simulink model "iC_1ph_MR2_0829"  (Simulink 7.5)
settings: Solver=ode14x  StartTime=0.0  StopTime=30/60  FixedStep=Ts1  RelTol=1e-3
PostLoadFcn:
  | , if any(exist('dsrtsu_mdlpostloadfcn', 'file') == [2, 3, 6]), try dsrtsu_mdlpostloadfcn('Execute', bdroot); catch fprintf('Error in PostLoadFcn (dsrtsu_mdlpostloadfcn) for model "%s":\n %s\n', bdroot, lasterr); end, end,
InitFcn:
  | iC_ini
values from neighbouring files (symbols this model uses):
  C = Cideal+deltaC    (= 4e-05)    [IMC_calculo_limites_thetas.m]    (also in IMC_ini.m; JORGE_controlador_LCL_malha_interna.m; LCL_PAPM.m; R_in_LCL.m)
  excitacao_persistente = 0    [iC_ini.m]    (also in vC_ini.m)
  flag_time = 60/60    (= 1)    [iC_ini.m]    (also in vC_ini.m)
  init_time = 60/60    (= 1)    [iC_ini.m]
  L1 = L1ideal+deltaL1    (= 0.002)    [IMC_calculo_limites_thetas.m]    (also in IMC_ini.m; LCL_PAPM.m; R_in_LCL.m; calculo_FTs.m)
  L2 = L2ideal+deltaL2+Lgideal+deltaLg    (= 0.002)    [IMC_calculo_limites_thetas.m]    (also in IMC_ini.m; LCL_PAPM.m; R_in_LCL.m; calculo_FTs.m)
  param_change_time = 60/60    (= 1)    [iC_ini.m]    (also in vC_ini.m = 10)
  R1 = R1ideal+deltaR1    (= 1)    [IMC_calculo_limites_thetas.m]    (also in IMC_ini.m; R_in_LCL.m = 0; gera_resultados.m = 0; iC_ini.m = 0)
  R2 = R2ideal+deltaR2+Rgideal+deltaRg    (= 1)    [IMC_calculo_limites_thetas.m]    (also in IMC_ini.m; R_in_LCL.m = 0; gera_resultados.m = 0; iC_ini.m = 0)
  R_init = 10    [iC_ini.m]
  ref_phaseInv_time = 60/60    (= 1)    [iC_ini.m]    (also in vC_ini.m = 3.33333333333)
  ref_step_time = 60/60    (= 1)    [iC_ini.m]    (also in vC_ini.m = 6.66666666667)
  Ts = 1/12000    (= 8.33333333333e-05)    [IMC_calculo_limites_thetas.m]    (also in IMC_datta_ini.m = 0.5; IMC_ini.m; JORGE_controlador_LCL_malha_interna.m; LCL_PAPM.m)
  Ts1 = Ts/10    (= 8.33333333333e-06)    [iC_ini.m]    (also in vC_ini.m = 8.33333333333e-08)
  VCC = 1700    [iC_ini.m]    (also in vC_ini.m = 1200)
libraries: powerlib x14, powerlib_extras x1
settings Model: DSRTSU_INTERNAL_RTI_VER=390  DSRTSU_INTERNAL_RTI_TYPE=rti1103  Creator=dpbernardon  LastModifiedBy=dpbernardon  BufferReuse=off
settings SolverCC: AutoInsertRateTranBlk=on
settings OptimizationCC: BlockReduction=off  OptimizeBlockIOStorage=off  BufferReuse=off  ExpressionFolding=off  LocalBlockOutputs=off
settings HardwareCC: ProdIntDivRoundTo=Zero  ProdEndianess=BigEndian  ProdHWDeviceType=Generic->Custom  TargetIntDivRoundTo=Zero  TargetEndianess=BigEndian  TargetHWDeviceType=Generic->Custom
settings RTWCC: SystemTargetFile=rti1103.tlc  MakeCommand=make_rti  TemplateMakefile=rti1103.tmf  Description=dSPACE DS1103 Hardware Platform  ProcessScript=rti1103_make_rtw_hook
settings STFCustomTargetCC: ParMdlRefBuildCompliant=on  GeneratePreprocessorConditionals=Disable all  MatFileLogging=on  SystemTargetFile=rti1103.tlc
settings GRTTargetCC: CompOptLevelCompliant=off  ExtModeMexFile=noextcomm
settings CustomProperty: DataType=RTWOptions_EnumType_C__dSPACE RCPHIL 72_matlab_rti1103_tlc_rti1103_1InitialSimState  Value=RUN
settings EnumStrPairs: String=RUN

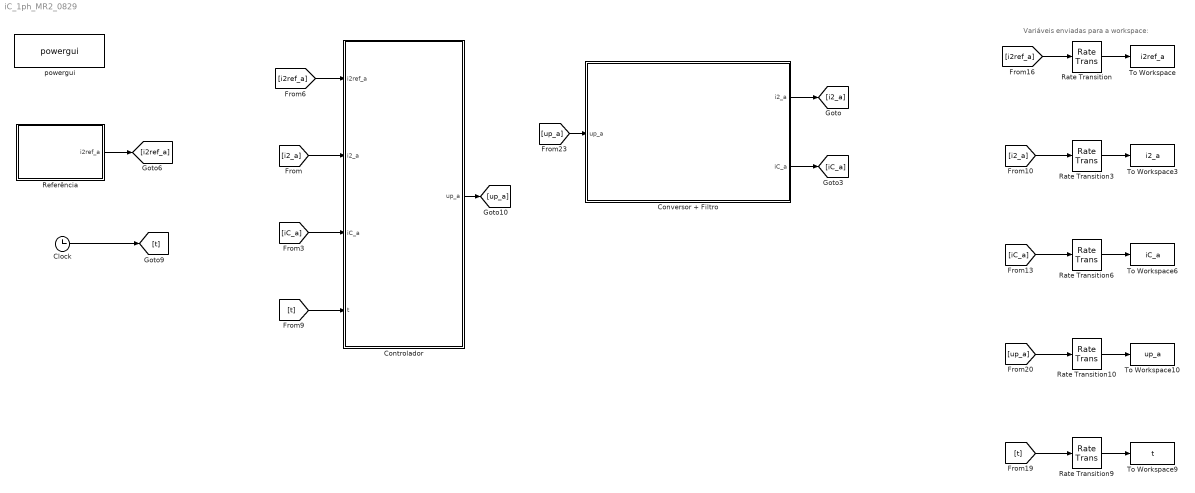
== system iC_1ph_MR2_0829 ==
  note: Variáveis enviadas para a workspace:
  Clock : Clock
      settings: Decimation=10
  Controlador : Subsystem
  Conversor + Filtro : Subsystem
  Rate Transition{,3,6,9..10} (5 alike) : RateTransition  OutPortSampleTime=Ts1
  Referência : Subsystem
  To Workspace : ToWorkspace  VariableName=i2ref_a  SampleTime=Ts1  SaveFormat=Array
  To Workspace10 : ToWorkspace  VariableName=up_a  SampleTime=Ts1  SaveFormat=Array
  To Workspace3 : ToWorkspace  VariableName=i2_a  SampleTime=Ts1  SaveFormat=Array
  To Workspace6 : ToWorkspace  VariableName=iC_a  SampleTime=Ts1  SaveFormat=Array
  To Workspace9 : ToWorkspace  VariableName=t  SampleTime=Ts1  SaveFormat=Array
  powergui : powerlib/powergui  Priority=1  SystemSampleTime=-1  SimulationMode=Discrete  SampleTime=Ts1  frequency=60  SPID=off  DisableSnubberDevices=off  DisableRonSwitches=off  DisableVfSwitches=off  SwTol=0  Interpol=off  frequencyindice=0  echomessages=off  HookPort=off  DisplayEquations=off  FunctionMessages=off  EnableUseOfTLC=off  x0status=blocks  RestoreLinks=warning  ResistiveCurrentMeasurement=off  Frange=[0:2:500]  Ylog=off  Xlog=on  ShowGrid=off  save=off  variable=ZData  ZoomFFT=off  StartTime=0.0  cycles=1  DisplayStyle=1  fundamental=60  FreqAxis=off  MaxFrequency=1000  frequencyindicesteady=1  RmsSteady=1  display=off  Ts=0  methode=off
  wires:
  Conversor + Filtro/1(i2_a) -> [i2_a]
  Conversor + Filtro/2(iC_a) -> [iC_a]
  [i2_a] -> Controlador/2(i2_a)
  [iC_a] -> Controlador/3(iC_a)
  Referência/1(i2ref_a) -> [i2ref_a]
  [i2ref_a] -> Controlador/1(i2ref_a)
  Clock/1 -> [t]
  [t] -> Controlador/4(t)
  [i2ref_a] -> Rate Transition/1
  [i2_a] -> Rate Transition3/1
  [iC_a] -> Rate Transition6/1
  [t] -> Rate Transition9/1
  Rate Transition/1 -> To Workspace/1
  Rate Transition3/1 -> To Workspace3/1
  Rate Transition6/1 -> To Workspace6/1
  Rate Transition9/1 -> To Workspace9/1
  [up_a] -> Rate Transition10/1
  Rate Transition10/1 -> To Workspace10/1
  Controlador/1(up_a) -> [up_a]
  [up_a] -> Conversor + Filtro/1(up_a)

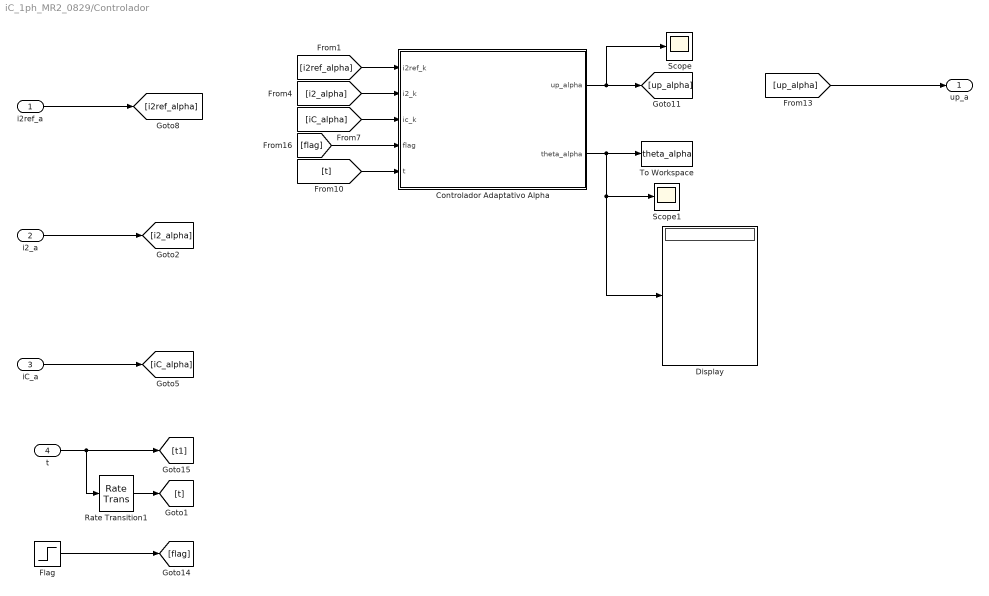
== system iC_1ph_MR2_0829/Controlador ==
  i2ref_a : Inport
  i2_a : Inport  Port=2
  iC_a : Inport  Port=3
  t : Inport  Port=4
  Controlador Adaptativo Alpha : Stateflow chart  TreatAsAtomicUnit=on  SystemSampleTime=Ts
      settings: MinAlgLoopOccurrences=on  RTWSystemCode=Function
  Display : Display
  Flag : Step  Time=flag_time  Before=1  After=0  SampleTime=Ts
  Rate Transition1 : RateTransition  OutPortSampleTime=Ts
  Scope : Scope
      settings: YMin=-5500  YMax=5000  SaveName=ScopeData4
  Scope1 : Scope
      settings: YMin=-5500  YMax=5000
  To Workspace : ToWorkspace  VariableName=theta_alpha  SampleTime=Ts1  SaveFormat=Array
  up_a : Outport
  wires:
  t/1 -> Rate Transition1/1, [t1]
  Rate Transition1/1 -> [t]
  i2_a/1 -> [i2_alpha]
  iC_a/1 -> [iC_alpha]
  [i2ref_alpha] -> Controlador Adaptativo Alpha/1(i2ref_k)
  [i2_alpha] -> Controlador Adaptativo Alpha/2(i2_k)
  [iC_alpha] -> Controlador Adaptativo Alpha/3(ic_k)
  [t] -> Controlador Adaptativo Alpha/5(t)
  Controlador Adaptativo Alpha/1(up_alpha) -> [up_alpha], Scope/1
  [up_alpha] -> up_a/1
  Flag/1 -> [flag]
  [flag] -> Controlador Adaptativo Alpha/4(flag)
  Controlador Adaptativo Alpha/2(theta_alpha) -> To Workspace/1, Scope1/1, Display/1
  i2ref_a/1 -> [i2ref_alpha]

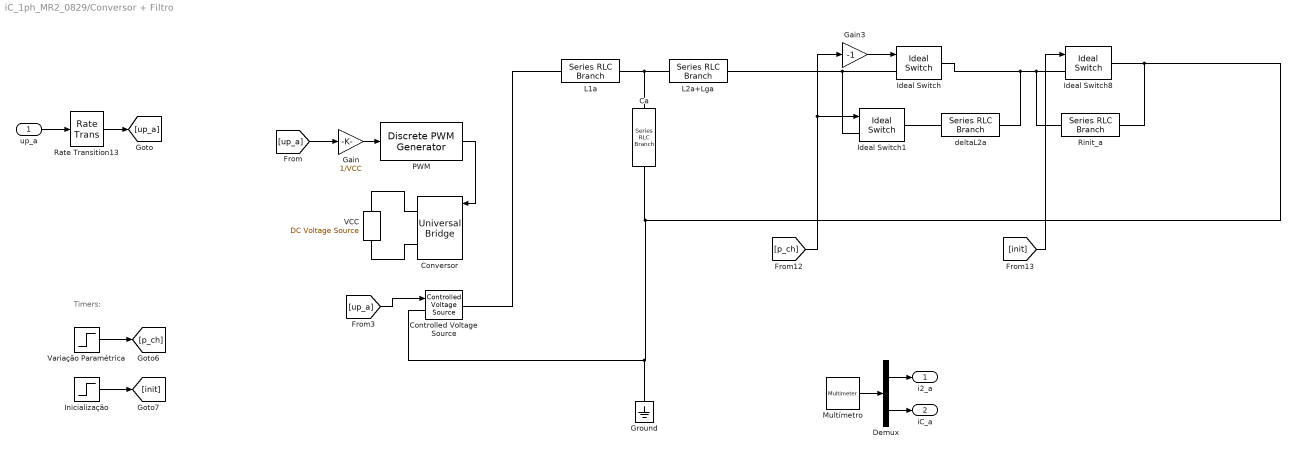
== system iC_1ph_MR2_0829/Conversor + Filtro ==
  note: Timers:
  up_a : Inport
  Ca : powerlib/Elements/Series RLC Branch  DialogController=POWERSYS.PowerSysDialog  PhysicalDomain=powersysdomain  SubClassName=unknown  LeftPortType=p1  RightPortType=p1  LConnTagsString=__new0  RConnTagsString=__new0  BranchType=C  Resistance=1  Inductance=1e-3  SetiL0=off  InitialCurrent=0  Capacitance=C  Setx0=off  InitialVoltage=0  Measurements=Branch current
  Controlled Voltage Source : powerlib/Electrical Sources/Controlled Voltage Source  DialogController=POWERSYS.PowerSysDialog  SystemSampleTime=-1  Initialize=on  Source_Type=AC  Amplitude=0  Phase=0  Frequency=0  Measurements=None
  Conversor : powerlib/Power Electronics/Universal Bridge  DialogController=POWERSYS.PowerSysDialog  SystemSampleTime=-1  Arms=3  SnubberResistance=1e5  SnubberCapacitance=inf  Device=IGBT / Diodes  Ron=1e-3  Lon=0  ForwardVoltages="[  0  0  ]"  ForwardVoltage=0  GTOparameters=[ 10e-6 , 20e-6 ]  IGBTparameters=[ 1e-6 , 2e-6 ]  Measurements=UAB UBC UCA UDC voltages  Measurements_2=None  converterType=Rectifier
  Demux : Demux  Outputs=2
  Gain : Gain  Gain=1/VCC  SampleTime=Ts1
  Gain3 : Gain  Gain=-1  SampleTime=Ts1
  Ground : powerlib/Elements/Ground  DialogController=POWERSYS.PowerSysDialog  PhysicalDomain=powersysdomain  SubClassName=unknown  LeftPortType=p1  RightPortType=p1  LConnTagsString=a
  Ideal Switch : powerlib/Power Electronics/Ideal Switch  DialogController=POWERSYS.PowerSysDialog  SystemSampleTime=-1  Ron=0.001  Lon=0  IC=1  Rs=1e5  Cs=inf  Measurements=off
  Ideal Switch1 : powerlib/Power Electronics/Ideal Switch  DialogController=POWERSYS.PowerSysDialog  SystemSampleTime=-1  Ron=0.001  Lon=0  IC=0  Rs=1e5  Cs=inf  Measurements=off
  Ideal Switch8 : powerlib/Power Electronics/Ideal Switch  DialogController=POWERSYS.PowerSysDialog  SystemSampleTime=-1  Ron=0.001  Lon=0  IC=1  Rs=1e5  Cs=inf  Measurements=off
  Inicialização : Step  Time=init_time  Before=1  After=0  SampleTime=Ts1
  L1a : powerlib/Elements/Series RLC Branch  DialogController=POWERSYS.PowerSysDialog  PhysicalDomain=powersysdomain  SubClassName=unknown  LeftPortType=p1  RightPortType=p1  LConnTagsString=__new0  RConnTagsString=__new0  BranchType=RL  Resistance=R1  Inductance=L1  SetiL0=off  InitialCurrent=0  Capacitance=1e-6  Setx0=off  InitialVoltage=0  Measurements=Branch current
  L2a+Lga : powerlib/Elements/Series RLC Branch  DialogController=POWERSYS.PowerSysDialog  PhysicalDomain=powersysdomain  SubClassName=unknown  LeftPortType=p1  RightPortType=p1  LConnTagsString=__new0  RConnTagsString=__new0  BranchType=RL  Resistance=R2  Inductance=L2  SetiL0=off  InitialCurrent=0  Capacitance=1e-6  Setx0=off  InitialVoltage=0  Measurements=Branch current
  Multímetro : powerlib/Measurements/Multimeter  SystemSampleTime=-1  PhasorSimulation=off  OutputType=Complex  sel=[7 5]  L=7  Gain=[1 1]  yselected={'Ib: Conversor + Filtro/L2a+Lga','Ib: Conversor + Filtro/Ca'};  PSBOutputType=1  PSBequivalent=0  AxesSetting=[0,0.1,-100,100]  Display=0  SavedBlockNames=-11
  PWM : powerlib_extras/Discrete  Control Blocks/Discrete PWM Generator  DialogController=POWERSYS.PowerSysDialog  SystemSampleTime=-1  GeneratorMode="3-arm  bridge (6 pulses)"  Fc=12000  Ts=Ts1  Internal=off  mIndex=0.4  Freq=60  Phase=0
  Rate Transition13 : RateTransition  OutPortSampleTime=Ts1
  Rinit_a : powerlib/Elements/Series RLC Branch  DialogController=POWERSYS.PowerSysDialog  PhysicalDomain=powersysdomain  SubClassName=unknown  LeftPortType=p1  RightPortType=p1  LConnTagsString=__new0  RConnTagsString=__new0  BranchType=RL  Resistance=R_init  Inductance=5*L2  SetiL0=off  InitialCurrent=0  Capacitance=1e-6  Setx0=off  InitialVoltage=0  Measurements=None
  VCC : powerlib/Electrical Sources/DC Voltage Source  DialogController=POWERSYS.PowerSysDialog  SystemSampleTime=-1  Amplitude=VCC  Measurements=None
  Variação Paramétrica : Step  Time=param_change_time  Before=-1  SampleTime=Ts1
  deltaL2a : powerlib/Elements/Series RLC Branch  DialogController=POWERSYS.PowerSysDialog  PhysicalDomain=powersysdomain  SubClassName=unknown  LeftPortType=p1  RightPortType=p1  LConnTagsString=__new0  RConnTagsString=__new0  BranchType=RL  Resistance=0  Inductance=5*L2  SetiL0=off  InitialCurrent=0  Capacitance=1e-6  Setx0=off  InitialVoltage=0  Measurements=None
  i2_a : Outport
  iC_a : Outport  Port=2
  wires:
  Gain/1 -> PWM/1
  up_a/1 -> Rate Transition13/1
  Rate Transition13/1 -> [up_a]
  PWM/1 -> Conversor/1
  [up_a] -> Gain/1
  [up_a] -> Controlled Voltage Source/1
  Multímetro/1 -> Demux/1
  Demux/1 -> i2_a/1
  Variação Paramétrica/1 -> [p_ch]
  Gain3/1 -> Ideal Switch/1
  [init] -> Ideal Switch8/1
  Inicialização/1 -> [init]
  [p_ch] -> Gain3/1, Ideal Switch1/1
  Demux/2 -> iC_a/1
  connections:
  Ideal Switch/RConn1 -- deltaL2a/RConn1 -- Ideal Switch8/LConn1 -- Rinit_a/LConn1
  Ca/LConn1 -- L2a+Lga/LConn1 -- L1a/RConn1
  Conversor/RConn1 -- VCC/RConn1
  VCC/LConn1 -- Conversor/RConn2
  L2a+Lga/RConn1 -- Ideal Switch/LConn1 -- Ideal Switch1/LConn1
  deltaL2a/LConn1 -- Ideal Switch1/RConn1
  Rinit_a/RConn1 -- Ideal Switch8/RConn1 -- Ground/LConn1 -- Controlled Voltage Source/LConn1 -- Ca/RConn1
  Controlled Voltage Source/RConn1 -- L1a/LConn1

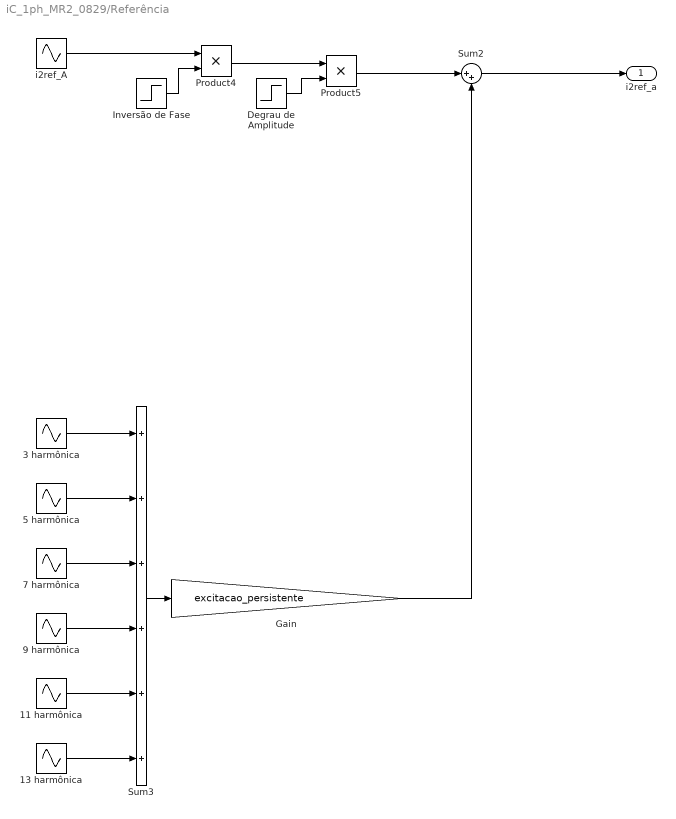
== system iC_1ph_MR2_0829/Referência ==
  11 harmônica : Sin  Amplitude=1.2  Bias=0  Frequency=2*pi*60*11  Phase=0  Samples=10  SampleTime=Ts  Offset=0
  13 harmônica : Sin  Amplitude=1.2  Bias=0  Frequency=2*pi*60*13  Phase=0  Samples=10  SampleTime=Ts  Offset=0
  3 harmônica : Sin  Amplitude=1.2  Bias=0  Frequency=2*pi*60*3  Phase=0  Samples=10  SampleTime=Ts  Offset=0
  5 harmônica : Sin  Amplitude=1.2  Bias=0  Frequency=2*pi*60*5  Phase=0  Samples=10  SampleTime=Ts  Offset=0
  7 harmônica : Sin  Amplitude=1.2  Bias=0  Frequency=2*pi*60*7  Phase=0  Samples=10  SampleTime=Ts  Offset=0
  9 harmônica : Sin  Amplitude=1.2  Bias=0  Frequency=2*pi*60*9  Phase=0  Samples=10  SampleTime=Ts  Offset=0
  Degrau de Amplitude : Step  Time=ref_step_time  Before=1  After=2  SampleTime=Ts
  Gain : Gain  Gain=excitacao_persistente  SampleTime=Ts
  Inversão de Fase : Step  Time=ref_phaseInv_time  Before=1  After=-1  SampleTime=Ts
  Product4 : Product  SampleTime=Ts  RndMeth=Zero
  Product5 : Product  SampleTime=Ts  RndMeth=Zero
  Sum2 : Sum  Inputs=|++
  Sum3 : Sum  Inputs=++++++
  i2ref_A : Sin  Amplitude=2  Bias=0  Frequency=2*pi*60  Phase=0  Samples=10  SampleTime=Ts  Offset=0
  i2ref_a : Outport
  wires:
  Product4/1 -> Product5/1
  Inversão de Fase/1 -> Product4/2
  Degrau de Amplitude/1 -> Product5/2
  i2ref_A/1 -> Product4/1
  Product5/1 -> Sum2/1
  Gain/1 -> Sum2/2
  Sum2/1 -> i2ref_a/1
  3 harmônica/1 -> Sum3/1
  5 harmônica/1 -> Sum3/2
  7 harmônica/1 -> Sum3/3
  9 harmônica/1 -> Sum3/4
  11 harmônica/1 -> Sum3/5
  13 harmônica/1 -> Sum3/6
  Sum3/1 -> Gain/1

== matlab function Controlador/Controlador Adaptativo Alpha ==
  data: i2ref_k input double; up_alpha output double; i2_k input double; ic_k input double; flag input double; t input double; theta_alpha output double
function [up_alpha,theta_alpha] = adaptativo( i2ref_k, i2_k, ic_k, flag, t )

%#CODEGEN
    
%Definição dos valores projetados dos elementos do filtro
L1ideal=2e-3;
L2ideal=2e-3;
Lgideal=0;
Cideal=40e-6;
R1ideal=0;
R2ideal=0;
Rgideal=0;

%Definição de erros percentuais para simular variação paramétrica
errL1=0;
errL2=0;
errLg=0;
errC=0;
errR1=0;
errR2=0;
errRg=0;
deltaL1=errL1*L1ideal;
deltaL2=errL2*L2ideal;
deltaLg=errLg*Lgideal;
deltaC=errC*Cideal;
deltaR1=errR1*R1ideal;
deltaR2=errR2*R2ideal;
deltaRg=errRg*Rgideal;

%Definição do valor real medido, incluindo a variação paramétrica
%percentual
L1=L1ideal+deltaL1;
L2=L2ideal+deltaL2+Lgideal+deltaLg;
C=Cideal+deltaC;
R1=R1ideal+deltaR1;
R2=R2ideal+deltaR2+Rgideal+deltaRg;

%Demais elementos
Ts=1/12000;
w=sqrt((L1+L2)/(L1*L2*C));

%Kp é a multiplicação do ganho do controlador da malha interna(kp), do
%ganho da planta(ki) e do ganho da malha externa(kod)
kp=8;
%Kp=0.156891976007044;
Kp=0.004780841242217;

%polos do modelo de referência:
p1=0.2;
p2=0.2;

km=(1-p1)*(1-p2);

%constantes -> gamaD < (1-gama)*km/kp
gamaD=0.0098;
gama=0.99;

delta0=0.8;

%adapt_time=2/60;
%vg_switch_time=4/60;

%if t>=19/60
%    stop=1;
%end

%% Variáveis Persistentes e Inicializações

persistent theta_k;
if isempty(theta_k)
    %COM compensação para vg
    %theta_k=[-0.3106; -0.2728; 0.0368; -0.2369; -0.422; -0.2775; -0.7979; 1.786; -0.0008; 0.0003];
    %theta_k=[-0.3106; -0.2728; 0.0368; -0.2369; -0.422; -0.2775; -0.7979; 1.786; 1; 0];
    %theta_k=[-0.40085038; -0.36853743; -0.064251891; -0.4277604154; -0.61214672; -0.46675405; -0.98929343; 1.76426551; 0.17164080; 0.11598547];
    %theta_k=[0;0;0;0;0;0; -0.98929343; 1.76426551; 0.17164080; 0.11598547];
    %theta_k=[-0.071151848470510; -0.470549298500393; -0.993323557655345; 1.762541193804541; 0.118014567931226; 0.108368323169129];
    %theta_k=[-0.46; -0.58; -1.74; 1.73; 0.2; 0.03];
    %theta_k=[-0.03; -0.36; -0.57; -0.01; 0.16; 0.02];
    theta_k=[0.34; -0.36; -0.51; 0.86; 0; 0];
end

persistent omega_k;
if isempty(omega_k)
    %COM vg
    omega_k=[0; 0; 0; 0; 0; 0];
end

persistent omega_k_1;
if isempty(omega_k_1)
    %COM vg
    omega_k_1=[0; 0; 0; 0; 0; 0];
end

persistent omega_k_2;
if isempty(omega_k_2)
    %COM vg
    omega_k_2=[0; 0; 0; 0; 0; 0];
end

%persistent omega_k_3;
%if isempty(omega_k_3)
%    %COM vg
%    omega_k_3=[0; 0; 0; 0; 0; 0];
%end

persistent eta_k_1;
if isempty(eta_k_1)
    %COM vg
    eta_k_1=[0; 0; 0; 0; 0; 0];
end

persistent eta_k_2;
if isempty(eta_k_2)
    %COM vg
    eta_k_2=[0; 0; 0; 0; 0; 0];
end

%persistent eta_k_3;
%if isempty(eta_k_3)
%    %COM vg
%    eta_k_3=[0; 0; 0; 0; 0; 0];
%end

persistent i2m_k_1;
if isempty(i2m_k_1)
    i2m_k_1=0;
end

persistent i2m_k_2;
if isempty(i2m_k_2)
    i2m_k_2=0;
end

%persistent i2m_k_3;
%if isempty(i2m_k_3)
%    i2m_k_3=0;
%end

persistent i2ref_k_1;
if isempty(i2ref_k_1)
    i2ref_k_1=0;
end

persistent i2ref_k_2;
if isempty(i2ref_k_2)
    i2ref_k_2=0;
end

%persistent i2ref_k_3;
%if isempty(i2ref_k_3)
%    i2ref_k_3=0;
%end

persistent v_k_1;
if isempty(v_k_1)
    v_k_1=0;
end

persistent v_k_2;
if isempty(v_k_2)
    v_k_2=0;
end

%persistent v_k_3;
%if isempty(v_k_3)
%    v_k_3=0;
%end

persistent rho_k;
if isempty(rho_k)
    rho_k=Kp/km;
end

persistent m2;
if isempty(m2)
    m2=1;
end

persistent u_k_1;
if isempty(u_k_1)
    u_k_1=0;
end

persistent u_k_2;
if isempty(u_k_2)
    u_k_2=0;
end

persistent P;
if isempty(P)
    %P=[0.002225441018075 -0.002258665319558 -1.129332659782590e-004 -0.003793046611769; ...
    %    -0.002258665319558 0.149747822133961 -0.042512608892738 0.002487914954665; ...
    %    -1.129332659782590e-004 -0.042512608892738 0.997874369555398 1.243957477280539e-004; ...
    %    -0.003793046611769 0.002487914954665 1.243957477280538e-004 0.754190018333160];
    %P=[0.009712540165252   -0.000020445335620  -0.000026266935611  -0.000037334327242 -0.001161097577207  -0.000971095497459; ...
    %   -0.000020445335620   0.009977400822109  -0.000022631160072  -0.000009984284241 -0.000310511239892   0.000028021469709; ...
    %   -0.000026266935611  -0.000022631160072   0.009976301443788  -0.000009972563160 -0.000310146714255   0.000019062507239; ...
    %   -0.000037334327242  -0.000009984284241  -0.000009972563160   0.009989966652248 -0.000312037115068   0.000004936266851; ...
    %   -0.001161097577207  -0.000310511239892  -0.000310146714255  -0.000312037115068 0.000295645721395   0.000153517899078; ...
    %   -0.000971095497459   0.000028021469709   0.000019062507239   0.000004936266851 0.000153517899078   0.000171767843043];

    P=gamaD*eye(6);
end

persistent gama2;
if isempty(gama2)
    %gama2=0.997899999973786;
    gama2=gama;
end

% persistent u_res_k1;
% if isempty(u_res_k1)
%     u_res_k1=0;
% end
% 
% persistent u_res_k2;
% if isempty(u_res_k2)
%     u_res_k2=0;
% end
% 
% persistent e_res_k1;
% if isempty(e_res_k1)
%     e_res_k1=0;
% end
% 
% persistent e_res_k2;
% if isempty(e_res_k2)
%     e_res_k2=0;
% end

%persistent adapt_init_flag;
%if isempty(adapt_init_flag)
%    adapt_init_flag=0;
%end

%if t>=adapt_time

%% Cálculos

%Ação de controle
omega_k(3)= i2_k;
omega_k(4)= i2ref_k;

%if t>vg_switch_time
%    omega_k(5)= 311*sin(2*pi*60*t);
%    omega_k(6)= 311*cos(2*pi*60*t);
%    if adapt_init_flag<1
%        theta_k(5)=0;
%        theta_k(6)=-1;
%        %theta_k=[0.3127; -0.3906; -0.7082; 1.0079; 0.0873; 0.0164;];
%        adapt_init_flag=1;
%    end
%else
%    omega_k(5)= 0;
%    omega_k(6)= 0;
%end

%omega_k(5)= 311*sin(2*pi*60*t);
%omega_k(6)= 311*cos(2*pi*60*t);

omega_k(5)= 0;
omega_k(6)= 0;

u_k= theta_k'*omega_k;

%inserindo o controlador proporcional no bloco do adaptativo
up_alpha= kp*(u_k-ic_k);

eta_k= (p1+p2)*eta_k_1 - p1*p2*eta_k_2 + (1-p1)*(1-p2)*omega_k_2;

i2m_k= (p1+p2)*i2m_k_1 - p1*p2*i2m_k_2 + (1-p1)*(1-p2)*i2ref_k_2;

e1_k= i2_k - i2m_k;

v_k= (p1+p2)*v_k_1 - p1*p2*v_k_2 + (1-p1)*(1-p2)*u_k_2;

q_k= theta_k'*eta_k;

e2_k= -v_k+q_k;

ea_k= e1_k+rho_k*e2_k;

if flag==1
    m2_k= 0.1*(eta_k'*eta_k) + e2_k^2 + m2;
else
    m2_k= 0.01*(eta_k'*eta_k) + e2_k^2 + m2;
end
%m2_k= m2 + (1+eta_k'*P*eta_k) + gama2*e2_k^2;

P= P - (P*(eta_k*eta_k')*P)/m2_k;
gama2= gama2 - (gama2^2*e2_k^2)/(m2_k^2);

%Pout=P;
%gama_out=gama2;

%% Atualização

%calcula theta(k+1)
theta_k = theta_k - (gamaD*ea_k/m2_k)*eta_k;
%theta_k = theta_k - (P*ea_k/m2_k)*eta_k;
theta_alpha = theta_k;

%calcula rho(k+1)
rho_k= rho_k - (gama*ea_k*e2_k)/m2_k;

if flag==1
    m2 = delta0*(m2 - 1) + abs(u_k) + abs(i2_k) + 1;
else
    m2 = delta0*(m2 - 1) + abs(u_k) + abs(i2_k) + 1;
end

%omega_k_3=omega_k_2;
omega_k_2=omega_k_1;
omega_k_1=omega_k;

omega_k(1)=0*omega_k(1) + 1*u_k;
omega_k(2)=0*omega_k(2) + 1*i2_k;

%eta_k_3=eta_k_2;
eta_k_2=eta_k_1;
eta_k_1=eta_k;

%i2ref_k_3 = i2ref_k_2;
i2ref_k_2 = i2ref_k_1;
i2ref_k_1 = i2ref_k;

%i2m_k_3=i2m_k_2;
i2m_k_2=i2m_k_1;
i2m_k_1=i2m_k;

%v_k_3=v_k_2;
v_k_2=v_k_1;
v_k_1=v_k;

u_k_2=u_k_1;
u_k_1=u_k;

%else

%e_res_k=0-ic_k;
%u_res_k= 1.98*u_res_k1 - u_res_k2 + 1.25*10^(-5)*(e_res_k1 - e_res_k2);

%up_alpha= kp*e_res_k + u_res_k;

%e_res_k2 = e_res_k1;
%e_res_k1 = e_res_k;
%u_res_k2 = u_res_k1;
%u_res_k1 = u_res_k;

%end

end
